simulink model "questao5"  (R2023a)
settings: Solver=VariableStepAuto  StartTime=0.0  StopTime=50  RelTol=1e-3
settings Model: Creator=franz  LastModifiedBy=franz

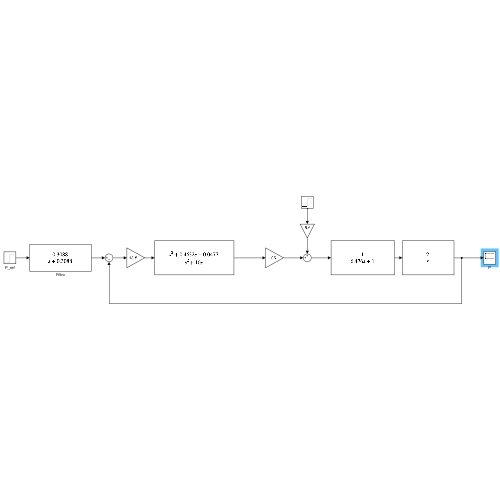
[thumbnail: Simulink's stored preview of the top-level diagram]
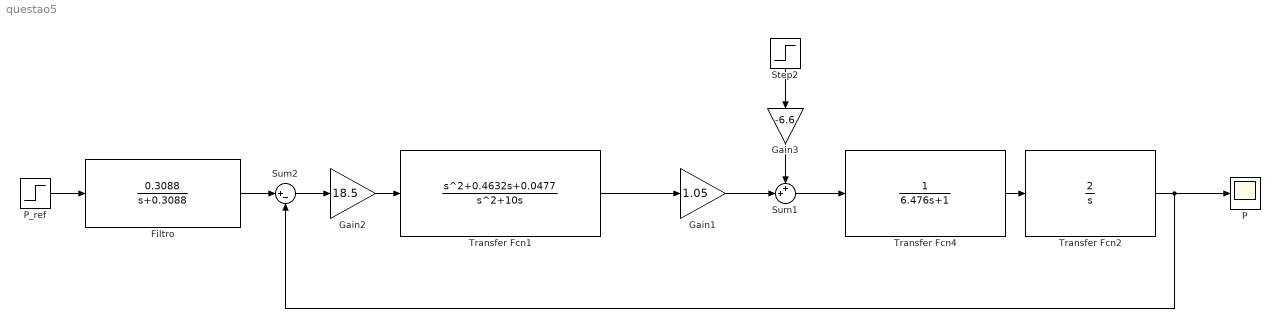
== system questao5 ==
  Filtro : TransferFcn  Numerator=[0.3088]  Denominator=[1 0.3088]
  Gain1 : Gain  Gain=1.05
  Gain2 : Gain  Gain=18.5
  Gain3 : Gain  Gain=-6.6
  P : Scope
  P_ref : Step  Time=10  After=50  SampleTime=0
  Step2 : Step  Time=30  After=0.25  SampleTime=0
  Sum1 : Sum  Inputs=++|
  Sum2 : Sum  Inputs=|+-
  Transfer Fcn1 : TransferFcn  Numerator=[1 0.4632 0.0477]  Denominator=[1 10 0]
  Transfer Fcn2 : TransferFcn  Numerator=[2]  Denominator=[1 0]
  Transfer Fcn4 : TransferFcn  Denominator=[6.476 1]
  wires:
  Filtro/1 -> Sum2/1
  P_ref/1 -> Filtro/1
  Transfer Fcn4/1 -> Transfer Fcn2/1
  Gain2/1 -> Transfer Fcn1/1
  Sum2/1 -> Gain2/1
  Transfer Fcn1/1 -> Gain1/1
  Gain1/1 -> Sum1/2
  Sum1/1 -> Transfer Fcn4/1
  Gain3/1 -> Sum1/1
  Step2/1 -> Gain3/1
  Transfer Fcn2/1 -> P/1, Sum2/2
